simulink model "microgrid_4DER"  (R2020a)
settings: Solver=VariableStepAuto  StartTime=0.0  StopTime=10.0  RelTol=1e-3
values from neighbouring files (symbols this model uses):
  cf1 = 50 * 1e-6    (= 5e-05)    [parameters.m]
  F1 = 0.75    [parameters.m]
  kic1 = 16e3    (= 16000)    [parameters.m]
  kiv1 = 390    [parameters.m]
  kpc1 = 10.5    [parameters.m]
  kpv1 = 0.05    [parameters.m]
  Lc1 = 0.35 * 1e-3    (= 0.00035)    [parameters.m]
  Lf1 = 1.35 * 1e-3    (= 0.00135)    [parameters.m]
  mp1 = 9.4 * 1e-5    (= 9.4e-05)    [parameters.m]
  nq1 = 1.3 * 1e-3    (= 0.0013)    [parameters.m]
  Rc1 = 0.03    [parameters.m]
  Rf1 = 0.1    [parameters.m]
  Tss = 2.5e-6    (= 2.5e-06)    [parameters.m]
  wb1 = 50 * 2 * pi    (= 314.159265359)    [parameters.m]
  wc1 = 31.41    [parameters.m]
  wcom = 0 * 2 * pi    (= 0)    [parameters.m]
undefined symbols (not defined in the file or in its folder): L11, L12, L13, Lf, R11, R12, R13
libraries: powerlib x46, powerlib_meascontrol x28
(part 2 of 2)

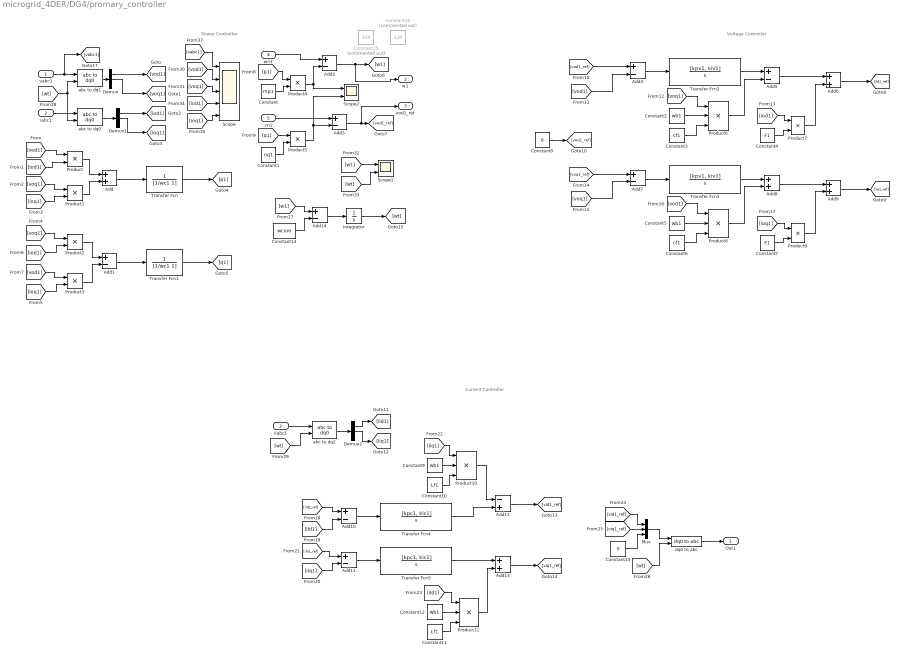
== system microgrid_4DER/DG4/promary_controller ==
  note: Voltage Controller
  note: Power Controller
  note: Current Controller
  vabc1 : Inport
  iabc1 : Inport  Port=2
  ilabc1 : Inport  Port=3
  wn1 : Inport  Port=4
  vn1 : Inport  Port=5
  Add{,6,8..9,13} (5 alike) : Sum
  Add{1..5,7,10..11,14} (9 alike) : Sum  Inputs=+-
  Add12 : Sum  Inputs=-+
  Constant : Constant  Value=mp1
  Constant1 : Constant  Value=nq1
  Constant10 : Constant  Value=Lf1
  Constant11 : Constant  Value=Lf1
  Constant{2,5,9,12} (4 alike) : Constant  Value=wb1
  Constant13 : Constant  Value=0
  Constant14 : Constant  Value=wcom  SampleTime=Tss
  Constant15 : Constant  Commented=on  Value=314
  Constant16 : Constant  Commented=on  Value=320
  Constant3 : Constant  Value=cf1
  Constant4 : Constant  Value=F1
  Constant6 : Constant  Value=cf1
  Constant7 : Constant  Value=F1
  Constant8 : Constant  Value=0
  Demux : Demux  Outputs=3
  Demux1 : Demux  Outputs=3
  Demux2 : Demux  Outputs=3
  Integrator : Integrator
  Mux : Mux  Inputs=3
  Product{,1..5,7,9} (8 alike) : Product
  Product{6,8,10..11} (4 alike) : Product  Inputs=3
  Scope : Scope  NumInputPorts=5
  Scope1 : Scope  NumInputPorts=2
  Scope2 : Scope  NumInputPorts=2
  Transfer Fcn : TransferFcn  Denominator=[1/wc1 1]
  Transfer Fcn1 : TransferFcn  Denominator=[1/wc1 1]
  Transfer Fcn2 : TransferFcn  Numerator=[kpv1, kiv1]  Denominator=[1, 0]
  Transfer Fcn3 : TransferFcn  Numerator=[kpv1, kiv1]  Denominator=[1, 0]
  Transfer Fcn4 : TransferFcn  Numerator=[kpc1, kic1]  Denominator=[1, 0]
  Transfer Fcn5 : TransferFcn  Numerator=[kpc1, kic1]  Denominator=[1, 0]
  abc to dq0 : powerlib_meascontrol/Transformations/abc to dq0  Alignment=90 degrees behind phase A axis
  abc to dq1 : powerlib_meascontrol/Transformations/abc to dq0  Alignment=90 degrees behind phase A axis
  abc to dq2 : powerlib_meascontrol/Transformations/abc to dq0  Alignment=90 degrees behind phase A axis
  dq0 to abc : powerlib_meascontrol/Transformations/dq0 to abc  Alignment=90 degrees behind phase A axis
  Out1 : Outport
  w1 : Outport  Port=2
  vod1_ref : Outport  Port=3
  wires:
  vabc1/1 -> [vabc1], abc to dq1/1
  iabc1/1 -> abc to dq0/1
  Demux/1 -> [vod1]
  Demux/2 -> [voq1]
  abc to dq1/1 -> Demux/1
  Demux1/2 -> [ioq1]
  Demux1/1 -> [iod1]
  abc to dq0/1 -> Demux1/1
  [vod1] -> Product/1
  [iod1] -> Product/2
  [voq1] -> Product1/1
  [ioq1] -> Product1/2
  Product/1 -> Add/1
  Product1/1 -> Add/2
  Add/1 -> Transfer Fcn/1
  Transfer Fcn/1 -> [p1]
  [voq1] -> Product2/1
  [iod1] -> Product2/2
  [vod1] -> Product3/1
  [ioq1] -> Product3/2
  Product2/1 -> Add1/1
  Product3/1 -> Add1/2
  Transfer Fcn1/1 -> [q1]
  Add1/1 -> Transfer Fcn1/1
  [p1] -> Product4/1
  Constant/1 -> Product4/2
  Product4/1 -> Scope2/1, Add2/2
  Add2/1 -> w1/1, [w1]
  [q1] -> Product5/1
  Constant1/1 -> Product5/2
  Product5/1 -> Scope2/2, Add3/2
  Add3/1 -> vod1_ref/1, [vod1_ref]
  [vod1_ref] -> Add4/1
  [vod1] -> Add4/2
  Add4/1 -> Transfer Fcn2/1
  Transfer Fcn2/1 -> Add5/1
  Constant2/1 -> Product6/2
  [voq1] -> Product6/1
  Constant3/1 -> Product6/3
  Product6/1 -> Add5/2
  Add5/1 -> Add6/1
  [iod1] -> Product7/1
  Constant4/1 -> Product7/2
  Product7/1 -> Add6/2
  Add6/1 -> [ild1_ref]
  Product8/1 -> Add8/2
  Constant6/1 -> Product8/3
  Add9/1 -> [ilq1_ref]
  Constant7/1 -> Product9/2
  Product9/1 -> Add9/2
  [ioq1] -> Product9/1
  Constant5/1 -> Product8/2
  [voq1] -> Add7/2
  [voq1_ref] -> Add7/1
  Add7/1 -> Transfer Fcn3/1
  Add8/1 -> Add9/1
  Transfer Fcn3/1 -> Add8/1
  [vod1] -> Product8/1
  Constant8/1 -> [voq1_ref]
  ilabc1/1 -> abc to dq2/1
  abc to dq2/1 -> Demux2/1
  Demux2/1 -> [ild1]
  Demux2/2 -> [ilq1]
  [ild1_ref] -> Add10/1
  [ild1] -> Add10/2
  [ilq1] -> Add11/2
  [ilq1_ref] -> Add11/1
  Add10/1 -> Transfer Fcn4/1
  Add11/1 -> Transfer Fcn5/1
  Transfer Fcn4/1 -> Add12/2
  [ilq1] -> Product10/1
  Constant9/1 -> Product10/2
  Constant10/1 -> Product10/3
  Product10/1 -> Add12/1
  Add12/1 -> [vid1_ref]
  Constant12/1 -> Product11/2
  [ild1] -> Product11/1
  Constant11/1 -> Product11/3
  Product11/1 -> Add13/2
  Transfer Fcn5/1 -> Add13/1
  Add13/1 -> [viq1_ref]
  [vid1_ref] -> Mux/1
  [viq1_ref] -> Mux/2
  Mux/1 -> dq0 to abc/1
  dq0 to abc/1 -> Out1/1
  [wt] -> dq0 to abc/2
  Constant13/1 -> Mux/3
  Constant14/1 -> Add14/2
  Add14/1 -> Integrator/1
  Integrator/1 -> [wt]
  [wt] -> abc to dq0/2, abc to dq1/2
  [wt] -> abc to dq2/2
  [w1] -> Scope1/1
  [wt] -> Scope1/2
  [ioq1] -> Scope/5
  [iod1] -> Scope/4
  [voq1] -> Scope/3
  [vod1] -> Scope/2
  [vabc1] -> Scope/1
  [w1] -> Add14/1
  vn1/1 -> Add3/1
  wn1/1 -> Add2/1

== system microgrid_4DER/DG4/secondary_controller ==
  w1 : Inport
  w_ref : Inport  Port=2
  vod1_ref : Inport  Port=3
  v_ref : Inport  Port=4
  Add15 : Sum  Inputs=+-
  Add16 : Sum  Inputs=+-
  Gain1 : Gain  Gain=-30
  Gain2 : Gain  Gain=-30
  Integrator1 : Integrator  InitialCondition=50*2*pi
  Integrator2 : Integrator  InitialCondition=220*sqrt(2)
  Scope3 : Scope  NumInputPorts=2
  wn1 : Outport
  vn1 : Outport  Port=2
  wires:
  Add16/1 -> Gain2/1
  w1/1 -> Add15/1
  Add15/1 -> Gain1/1
  vod1_ref/1 -> Add16/1
  v_ref/1 -> Add16/2
  Integrator1/1 -> wn1/1, Scope3/1
  Gain2/1 -> Integrator2/1
  Gain1/1 -> Integrator1/1
  w_ref/1 -> Add15/2
  Integrator2/1 -> vn1/1, Scope3/2
